simulink model "canode"  (R2024b)
settings: Solver=VariableStepAuto  StartTime=0.0  StopTime=100  RelTol=1e-3
settings Model: Creator=10537  LastModifiedBy=10537
settings SolverCC: AlgebraicLoopSolver=TrustRegion
settings DataIOCC: ReturnWorkspaceOutputs=off
settings DebuggingCC: UnconnectedInputMsg=warning  UnconnectedOutputMsg=warning  UnconnectedLineMsg=warning  ArithmeticOperatorsInVariantConditions=warning
settings ModelReferenceCC: EnableRefExpFcnMdlSchedulingChecks=on
settings SFSimCC: CustomCodeUndefinedFunction=UseInterfaceOnly
settings RTWCC: GPUComputeCapability=3.5

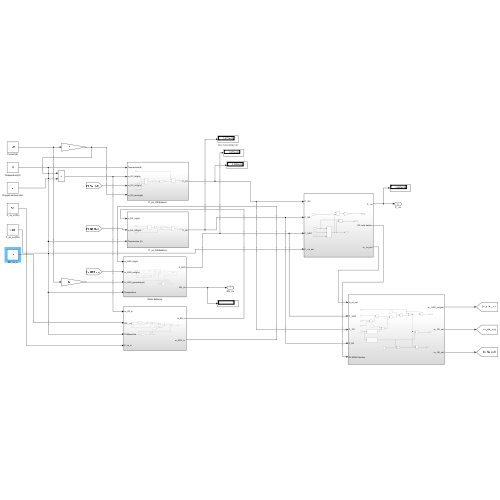
[thumbnail: Simulink's stored preview of the top-level diagram]
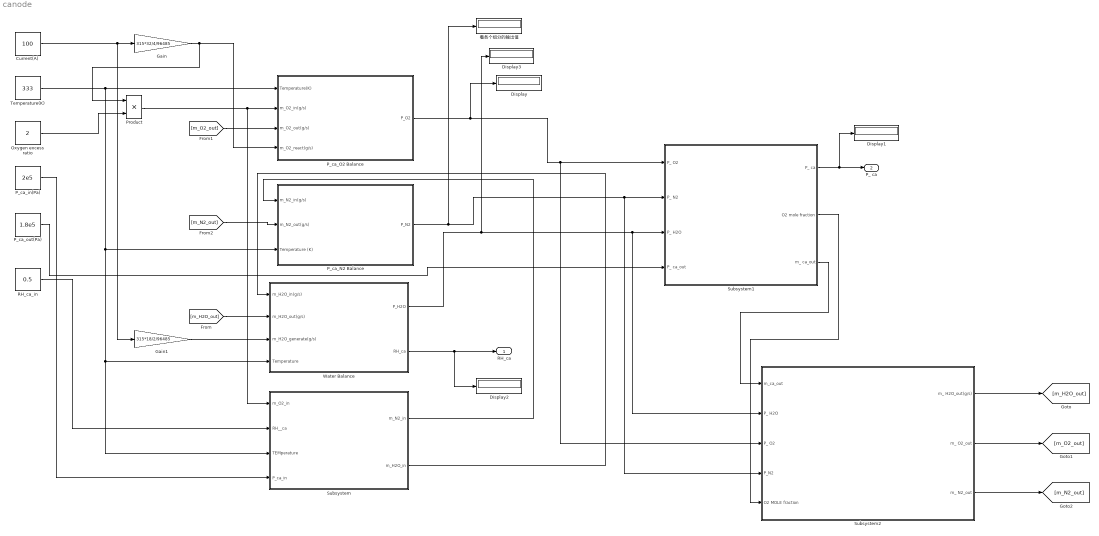
== system canode ==
  " P_ca_in(Pa) " : Constant  Value=2e5
  Current(A) : Constant  Value=100
  Display{,1..3} (4 alike) : Display
  Gain : Gain  Gain=315*32/4/96485
  Gain1 : Gain  Gain=315*18/2/96485
  "Oxygen excess ratio " : Constant  Value=2
  P_ca_N2 Balance : Subsystem
  P_ca_O2 Balance : Subsystem
  P_ca_out(Pa) : Constant  Value=1.8e5
  Product : Product
  RH_ca_in : Constant  Value=0.5
  Subsystem : Subsystem
  Subsystem1 : Subsystem
  Subsystem2 : Subsystem
  Temperature(K) : Constant  Value=333
  Water Balance : Subsystem
  看各个组分的输出值 : Display
  RH_ca : Outport  VectorParamsAs1DForOutWhenUnconnected=off
  P_ ca : Outport  Port=2
  wires:
  Temperature(K)/1 -> Subsystem/3(TEMperature), Water Balance/4("Temperature "), P_ca_N2 Balance/3(Temperature (K)), P_ca_O2 Balance/1(Temperature(K))
  Current(A)/1 -> Gain1/1, Gain/1
  Gain/1 -> Product/1, P_ca_O2 Balance/4(m_O2_react(g/s))
  "Oxygen excess ratio "/1 -> Product/2
  Product/1 -> Subsystem/1(m_O2_in), P_ca_O2 Balance/2(m_O2_in(g/s))
  Subsystem/2("m_H2O_in ") -> Water Balance/1(m_H2O_in(g/s))
  [m_H2O_out] -> Water Balance/2(m_H2O_out(g/s))
  Water Balance/1(P_H2O) -> Subsystem2/2(P_ H2O), Subsystem1/3(P_ H2O), Display3/1
  Water Balance/2(RH_ca) -> Display2/1, RH_ca/1
  Gain1/1 -> Water Balance/3(m_H2O_generate(g/s))
  RH_ca_in/1 -> Subsystem/2(RH__ca)
  " P_ca_in(Pa) "/1 -> Subsystem/4(P_ca_in)
  Subsystem/1(m_N2_in) -> P_ca_N2 Balance/1(m_N2_in(g/s))
  Subsystem1/1(P_ ca) -> Display1/1, P_ ca/1
  Subsystem1/3(m_ ca_out) -> Subsystem2/1(m_ca_out)
  P_ca_O2 Balance/1(P_O2) -> Display/1, Subsystem2/3(P_ O2), Subsystem1/1(P_ O2)
  P_ca_N2 Balance/1(P_N2) -> 看各个组分的输出值/1, Subsystem2/4(P_N2), Subsystem1/2(P_ N2)
  P_ca_out(Pa)/1 -> Subsystem1/4(P_ ca_out)
  Subsystem1/2(O2 mole fraction) -> Subsystem2/5(O2 MOLE fraction)
  Subsystem2/1(m_ H2O_out(g/s)) -> [m_H2O_out]
  Subsystem2/2(m_ O2_out) -> [m_O2_out]
  [m_O2_out] -> P_ca_O2 Balance/3(m_O2_out(g/s))
  Subsystem2/3(m_ N2_out) -> [m_N2_out]
  [m_N2_out] -> P_ca_N2 Balance/2(m_N2_out(g/s))

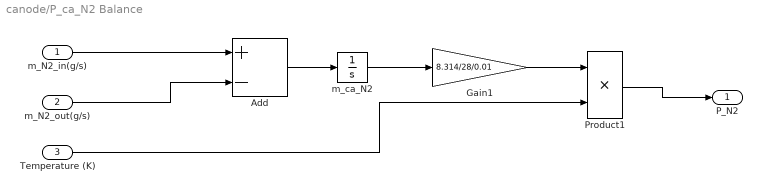
== system canode/P_ca_N2 Balance ==
  m_N2_in(g/s) : Inport
  m_N2_out(g/s) : Inport  Port=2
  Temperature (K) : Inport  Port=3
  Add : Sum  Inputs=+-
  Gain1 : Gain  Gain=8.314/28/0.01
  Product1 : Product
  m_ca_N2 : Integrator  InitialCondition=0.01
  P_N2 : Outport  VectorParamsAs1DForOutWhenUnconnected=off
  wires:
  Add/1 -> m_ca_N2/1
  m_N2_in(g/s)/1 -> Add/1
  m_N2_out(g/s)/1 -> Add/2
  Temperature (K)/1 -> Product1/2
  Gain1/1 -> Product1/1
  Product1/1 -> P_N2/1
  m_ca_N2/1 -> Gain1/1

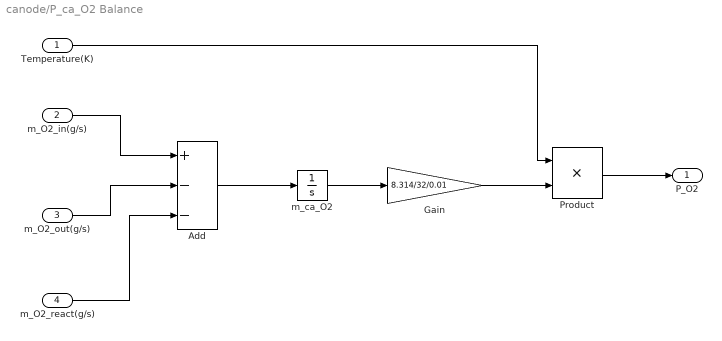
== system canode/P_ca_O2 Balance ==
  Temperature(K) : Inport
  m_O2_in(g/s) : Inport  Port=2
  m_O2_out(g/s) : Inport  Port=3
  m_O2_react(g/s) : Inport  Port=4
  Add : Sum  Inputs=+--
  Gain : Gain  Gain=8.314/32/0.01
  Product : Product
  m_ca_O2 : Integrator  InitialCondition=0.01
  P_O2 : Outport  VectorParamsAs1DForOutWhenUnconnected=off
  wires:
  Add/1 -> m_ca_O2/1
  m_O2_react(g/s)/1 -> Add/3
  m_O2_in(g/s)/1 -> Add/1
  m_ca_O2/1 -> Gain/1
  Product/1 -> P_O2/1
  Temperature(K)/1 -> Product/1
  Gain/1 -> Product/2
  m_O2_out(g/s)/1 -> Add/2

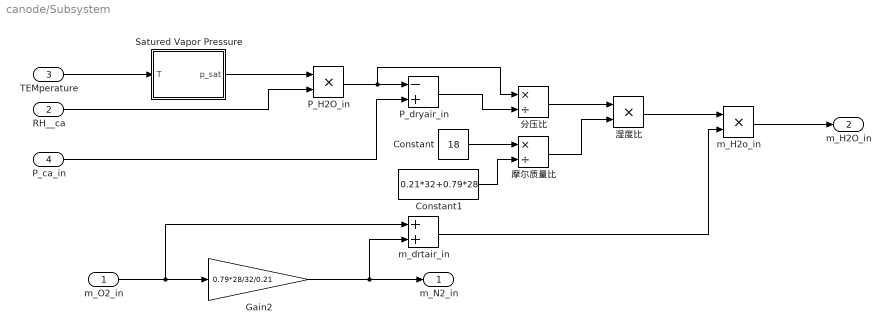
== system canode/Subsystem ==
  m_O2_in : Inport
  RH__ca : Inport  Port=2
  TEMperature : Inport  Port=3
  P_ca_in : Inport  Port=4
  Constant : Constant  Value=18
  Constant1 : Constant  Value=0.21*32+0.79*28
  Gain2 : Gain  Gain=0.79*28/32/0.21
  P_H2O_in : Product
  P_dryair_in : Sum  Inputs=-+
  "Satured Vapor Pressure " : MATLAB Function  TreatAsAtomicUnit=on
  "m_H2o_in " : Product
  m_drtair_in : Sum
  分压比 : Product  Inputs=*/
  摩尔质量比 : Product  Inputs=*/
  湿度比 : Product
  m_N2_in : Outport  VectorParamsAs1DForOutWhenUnconnected=off
  "m_H2O_in " : Outport  Port=2  VectorParamsAs1DForOutWhenUnconnected=off
  wires:
  TEMperature/1 -> "Satured Vapor Pressure "/1(T)
  P_ca_in/1 -> P_dryair_in/2
  Gain2/1 -> m_N2_in/1, m_drtair_in/2
  P_H2O_in/1 -> 分压比/1, P_dryair_in/1
  m_O2_in/1 -> m_drtair_in/1, Gain2/1
  Constant1/1 -> 摩尔质量比/2
  摩尔质量比/1 -> 湿度比/2
  湿度比/1 -> "m_H2o_in "/1
  m_drtair_in/1 -> "m_H2o_in "/2
  Constant/1 -> 摩尔质量比/1
  RH__ca/1 -> P_H2O_in/2
  P_dryair_in/1 -> 分压比/2
  "Satured Vapor Pressure "/1(p_sat) -> P_H2O_in/1
  "m_H2o_in "/1 -> "m_H2O_in "/1
  分压比/1 -> 湿度比/1

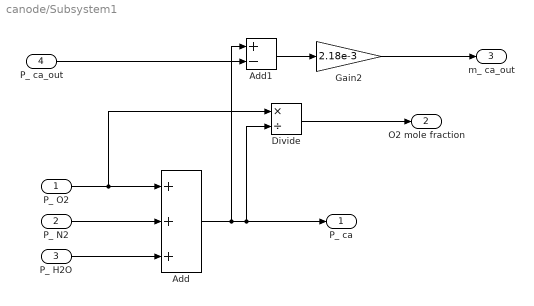
== system canode/Subsystem1 ==
  P_ O2 : Inport
  P_ N2 : Inport  Port=2
  P_ H2O : Inport  Port=3
  P_ ca_out : Inport  Port=4
  Add : Sum  Inputs=+++
  Add1 : Sum  Inputs=+-
  Divide : Product  Inputs=*/
  Gain2 : Gain  Gain=2.18e-3
  P_ ca : Outport
  O2 mole fraction : Outport  Port=2
  m_ ca_out : Outport  Port=3
  wires:
  Add1/1 -> Gain2/1
  Add/1 -> Add1/1, P_ ca/1, Divide/2
  P_ H2O/1 -> Add/3
  P_ N2/1 -> Add/2
  P_ ca_out/1 -> Add1/2
  Gain2/1 -> m_ ca_out/1
  P_ O2/1 -> Divide/1, Add/1
  Divide/1 -> O2 mole fraction/1

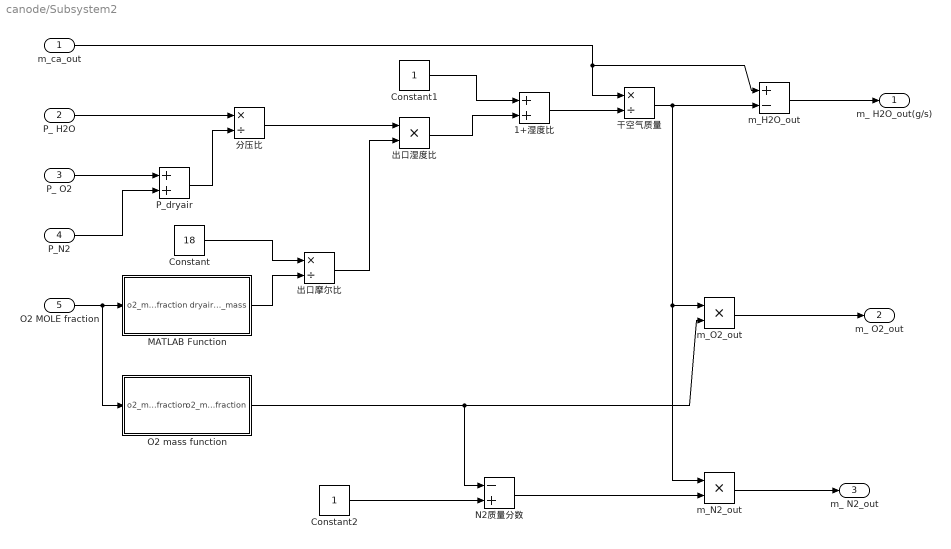
== system canode/Subsystem2 ==
  m_ca_out : Inport
  P_ H2O : Inport  Port=2
  P_ O2 : Inport  Port=3
  P_N2 : Inport  Port=4
  O2 MOLE fraction : Inport  Port=5
  1+湿度比 : Sum
  Constant : Constant  Value=18
  Constant1 : Constant
  Constant2 : Constant
  MATLAB Function : MATLAB Function  TreatAsAtomicUnit=on
  N2质量分数 : Sum  Inputs=-+
  O2 mass function : MATLAB Function  TreatAsAtomicUnit=on
  P_dryair : Sum
  m_H2O_out : Sum  Inputs=+-
  m_N2_out : Product
  m_O2_out : Product
  出口摩尔比 : Product  Inputs=*/
  出口湿度比 : Product
  分压比 : Product  Inputs=*/
  干空气质量 : Product  Inputs=*/
  m_ H2O_out(g/s) : Outport
  m_ O2_out : Outport  Port=2
  m_ N2_out : Outport  Port=3
  wires:
  P_dryair/1 -> 分压比/2
  m_ca_out/1 -> m_H2O_out/1, 干空气质量/1
  m_H2O_out/1 -> m_ H2O_out(g/s)/1
  出口摩尔比/1 -> 出口湿度比/2
  出口湿度比/1 -> 1+湿度比/2
  O2 mass function/1(o2_mass_fraction) -> N2质量分数/1, m_O2_out/2
  m_O2_out/1 -> m_ O2_out/1
  干空气质量/1 -> m_H2O_out/2, m_O2_out/1, m_N2_out/1
  P_N2/1 -> P_dryair/2
  N2质量分数/1 -> m_N2_out/2
  P_ O2/1 -> P_dryair/1
  1+湿度比/1 -> 干空气质量/2
  Constant2/1 -> N2质量分数/2
  P_ H2O/1 -> 分压比/1
  分压比/1 -> 出口湿度比/1
  O2 MOLE fraction/1 -> O2 mass function/1(o2_mole_fraction), MATLAB Function/1(o2_mole_fraction)
  MATLAB Function/1(dryair_mole_mass) -> 出口摩尔比/2
  Constant/1 -> 出口摩尔比/1
  Constant1/1 -> 1+湿度比/1
  m_N2_out/1 -> m_ N2_out/1

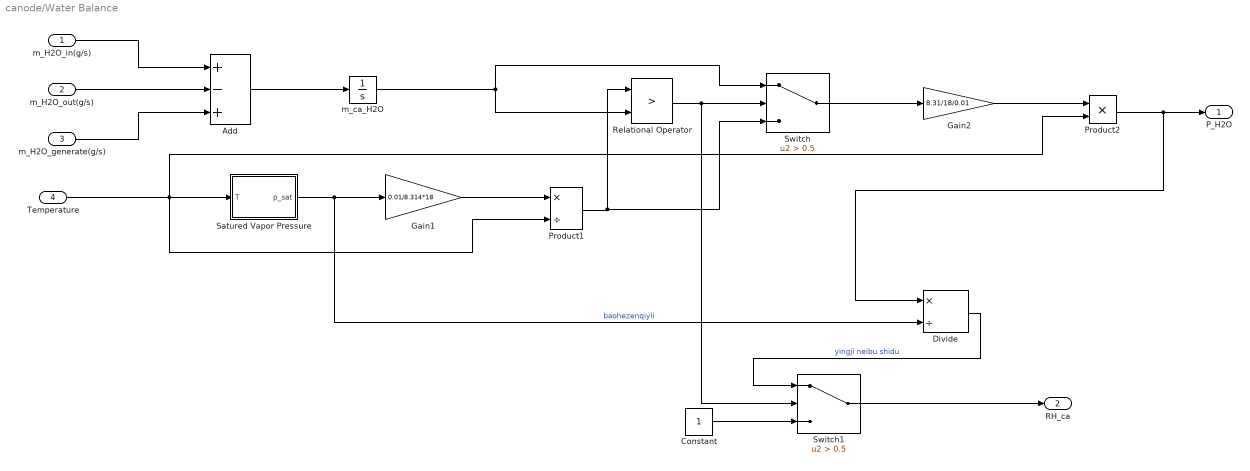
== system canode/Water Balance ==
  m_H2O_in(g/s) : Inport
  m_H2O_out(g/s) : Inport  Port=2
  m_H2O_generate(g/s) : Inport  Port=3
  "Temperature " : Inport  Port=4
  Add : Sum  Inputs=+-+
  Constant : Constant
  Divide : Product  Inputs=*/
  Gain1 : Gain  Gain=0.01/8.314*18
  Gain2 : Gain  Gain=8.31/18/0.01
  Product1 : Product  Inputs=*/
  Product2 : Product
  Relational Operator : RelationalOperator  Operator=>  OutDataTypeStr=boolean  RndMeth=Simplest  InputSameDT=off
  "Satured Vapor Pressure " : MATLAB Function  TreatAsAtomicUnit=on
  Switch : Switch  Criteria=u2 > Threshold  Threshold=0.5  SaturateOnIntegerOverflow=off  InputSameDT=off
  Switch1 : Switch  Criteria=u2 > Threshold  Threshold=0.5  SaturateOnIntegerOverflow=off  InputSameDT=off
  m_ca_H2O : Integrator  InitialCondition=0.01
  P_H2O : Outport  VectorParamsAs1DForOutWhenUnconnected=off
  RH_ca : Outport  Port=2  VectorParamsAs1DForOutWhenUnconnected=off
  wires:
  m_H2O_generate(g/s)/1 -> Add/3
  "Satured Vapor Pressure "/1(p_sat) -> Divide/2, Gain1/1  "baohezenqiyli"
  m_H2O_out(g/s)/1 -> Add/2
  m_ca_H2O/1 -> Relational Operator/2, Switch/1
  Product1/1 -> Switch/3, Relational Operator/1
  Constant/1 -> Switch1/3
  Add/1 -> m_ca_H2O/1
  Switch/1 -> Gain2/1
  Relational Operator/1 -> Switch1/2, Switch/2
  Product2/1 -> P_H2O/1, Divide/1
  Divide/1 -> Switch1/1  "yingji neibu shidu"
  m_H2O_in(g/s)/1 -> Add/1
  Gain1/1 -> Product1/1
  "Temperature "/1 -> Product2/2, Product1/2, "Satured Vapor Pressure "/1(T)
  Switch1/1 -> RH_ca/1
  Gain2/1 -> Product2/1

== matlab function canode/Water Balance/Satured Vapor Pressure  ==
  data: T input; p_sat output
function p_sat = fcn(T)%%求水的分压，饱和蒸汽压

p_sat = exp(23.196-3816.44/(T-46.13));

== matlab function canode/Subsystem2/MATLAB Function ==
  data: o2_mole_fraction input; dryair_mole_mass output
function dryair_mole_mass= fcn(o2_mole_fraction)

dryair_mole_mass = o2_mole_fraction*32+(1-o2_mole_fraction)*28;

== matlab function canode/Subsystem2/O2 mass function ==
  data: o2_mole_fraction input; o2_mass_fraction output
function o2_mass_fraction = fcn(o2_mole_fraction)

o2_mass_fraction =(o2_mole_fraction*32) /(o2_mole_fraction*32+(1-o2_mole_fraction)*28);

== matlab function canode/Subsystem/Satured Vapor Pressure  ==
  data: T input; p_sat output
function p_sat = fcn(T)%%求水的分压，饱和蒸汽压

p_sat = exp(23.196-3816.44/(T-46.13));
